simulink model "stepping_process"  (Simulink 3.00)
libraries: modellib x2

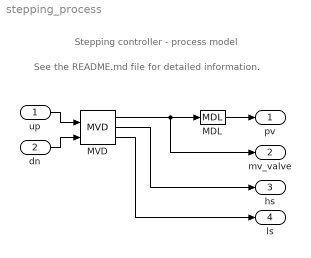
== system stepping_process ==
  note: See the README.md file for detailed information.
  note: Stepping controller - process model
  up : Inport  Port=1
  dn : Inport  Port=2
  MDL : modellib/MDL  k0=1  del=1  tau1=20  tau2=10  nmax=100
  MVD : modellib/MVD  y0=0  tv=10  hilim=1  lolim=0
  pv : Outport  Port=1
  mv_valve : Outport  Port=2
  hs : Outport  Port=3
  ls : Outport  Port=4
  wires:
  MDL/1 -> pv/1
  MVD/1 -> MDL/1, mv_valve/1
  MVD/2 -> hs/1
  MVD/3 -> ls/1
  dn/1 -> MVD/2
  up/1 -> MVD/1
